simulink model "PartA"  (R2024b)
settings: Solver=VariableStepAuto  StartTime=0.0  StopTime=10.0  RelTol=1e-3
settings Model: Creator=user  LastModifiedBy=user

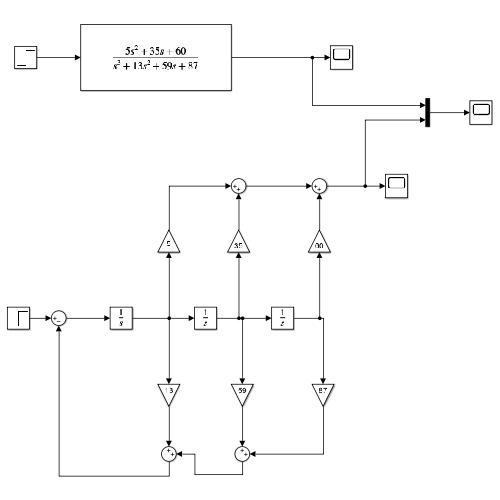
[thumbnail: Simulink's stored preview of the top-level diagram]
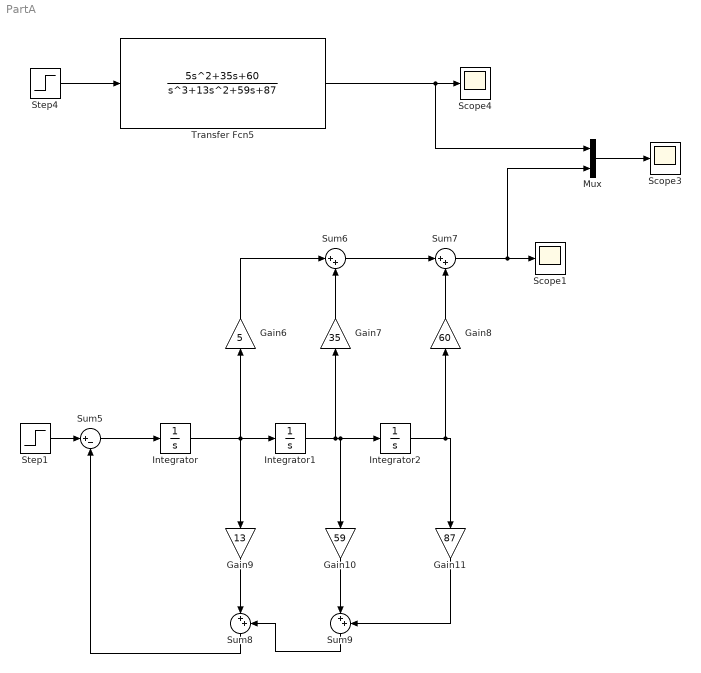
== system PartA ==
  Gain10 : Gain  Gain=59
  Gain11 : Gain  Gain=87
  Gain6 : Gain  Gain=5
  Gain7 : Gain  Gain=35
  Gain8 : Gain  Gain=60
  Gain9 : Gain  Gain=13
  Integrator : Integrator
  Integrator1 : Integrator
  Integrator2 : Integrator
  Mux : Mux  Inputs=2
  Scope1 : Scope
  Scope3 : Scope
  Scope4 : Scope
  Step1 : Step  Time=0  SampleTime=0
  Step4 : Step  Time=0  SampleTime=0
  Sum5 : Sum  Inputs=|+-
  Sum{6..9} (4 alike) : Sum  Inputs=|++
  Transfer Fcn5 : TransferFcn  Numerator=[5 35 60]  Denominator=[1 13 59 87]
  wires:
  Gain6/1 -> Sum6/1
  Sum7/1 -> Mux/2, Scope1/1
  Integrator/1 -> Integrator1/1, Gain9/1, Gain6/1
  Step1/1 -> Sum5/1
  Sum6/1 -> Sum7/1
  Sum8/1 -> Sum5/2
  Gain8/1 -> Sum7/2
  Integrator1/1 -> Gain7/1, Gain10/1, Integrator2/1
  Gain11/1 -> Sum9/2
  Sum5/1 -> Integrator/1
  Sum9/1 -> Sum8/2
  Gain9/1 -> Sum8/1
  Gain7/1 -> Sum6/2
  Integrator2/1 -> Gain11/1, Gain8/1
  Gain10/1 -> Sum9/1
  Mux/1 -> Scope3/1
  Step4/1 -> Transfer Fcn5/1
  Transfer Fcn5/1 -> Mux/1, Scope4/1
